simulink model "ARI_24_9_DBtracking"  (Simulink 7.8)
settings: Solver=ode45  SolverMode=SingleTasking  StartTime=0.0  StopTime=20  RelTol=1e-10  AbsTol=1e-10
values from neighbouring files (symbols this model uses):
  h = findobj(gcf,'type','line')    [boldLines.m]    (also in phase.m = min(hmax, 0.9*h*(tau/delta)^pow))
  p = plot(x,y,'b.',0,0,'g*','EraseMode','none','MarkerSize',10);hold on    [PAplot.m]
undefined symbols (not defined in the file or in its folder): A, B, C, D
libraries: simulink x9
settings Model: Creator=Michael Sebek  ModifiedByFormat=Michael Sebek  LastModifiedBy=Michael Sebek  ExtModeTrigMode=oneshot  ExtModeArmWhenConnect=off
settings DataIOCC: LimitDataPoints=off
settings OptimizationCC: BlockReduction=off  BooleanDataType=off  InitFltsAndDblsToZero=on
settings DebuggingCC: SaveWithParameterizedLinksMsg=none  SignalResolutionControl=TryResolveAllWithWarning  SolverPrmCheckMsg=none  MultiTaskDSMMsg=warning  MultiTaskCondExecSysMsg=none  FcnCallInpInsideContextMsg=Use local settings  StrictBusMsg=None
settings HardwareCC: TargetUnknown=on
settings RTWCC: IncludeERTFirstTime=on
settings GRTTargetCC: TargetFcnLib=ansi_tfl_tmw.mat

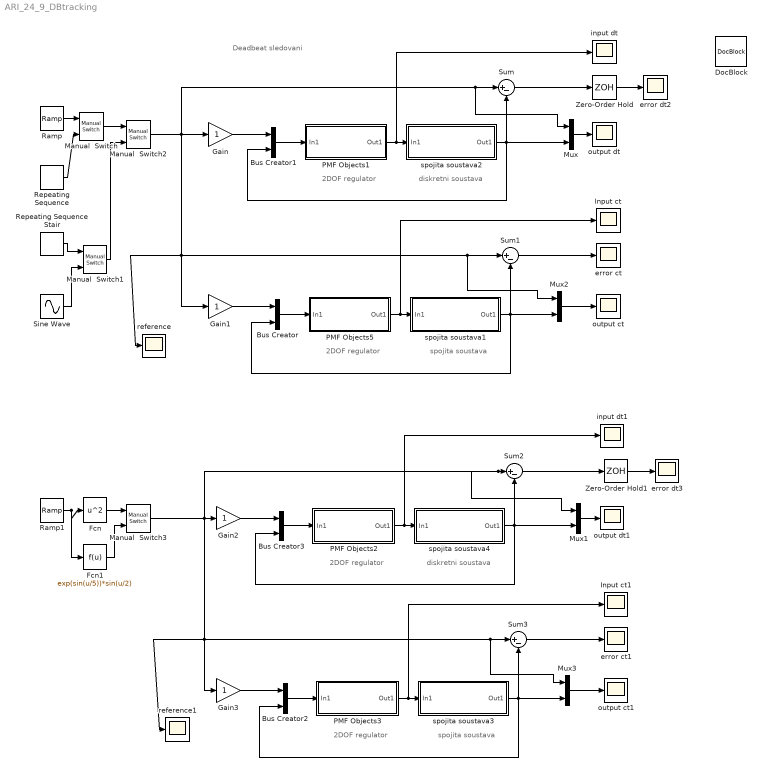
== system ARI_24_9_DBtracking ==
  note: Deadbeat sledovani
  note: spojita soustava
  note: 2DOF regulator
  note: diskretni soustava
  note: 2DOF regulator
  note: spojita soustava
  note: 2DOF regulator
  note: diskretni soustava
  note: 2DOF regulator
  Bus Creator{,1..3} (4 alike) : BusCreator  Inputs=2
  DocBlock : simulink/Model-Wide Utilities/DocBlock  DocumentType=Text
      content=|
      | %%%%%%%%%%%%%%%%%%%%%%%%%%%
      | sledovani rampy
      | %%%%%%%%%%%%%%%%%%%%%%%%%%%
      | h=0.5; m=1;f=(1-zi)^2;
      | a=(1-zi)^2;b=h^2/2*(zi+1)*zi;
      | [p,q]=axbyc(a,b,m);
      | [t,r]=axbyc(f,b,m);
      | p,q,t,r
      |
      | %%%%%%%%%%%%%%%%%%%%%%%%%%%
      | sledovani paraboly
      | %%%%%%%%%%%%%%%%%%%%%%%%%%%
      | h=0.5; m=1;f=(1-zi)^3;
      | a=(1-zi)^2;b=h^2/2*(zi+1)*zi;
      | [p,q]=axbyc(a,b,m);
      | [t,r]=axbyc(f,b,m);
      | p,q,t,r
  Fcn : Fcn  Expr=u^2
  Fcn1 : Fcn  Expr=exp(sin(u/5))*sin(u/2)
  Gain : Gain  SampleTime=h
  Gain1 : Gain
  Gain2 : Gain  SampleTime=h
  Gain3 : Gain
  Input ct : Scope
      settings: TickLabels=on  TimeRange=2  YMin=-2000  YMax=2000  DataFormat=Array
  Input ct1 : Scope
      settings: TickLabels=on  TimeRange=2  YMin=-2000  YMax=2000  SaveName=ScopeData7  DataFormat=Array
  Manual  Switch : simulink/Signal Routing/Manual Switch  sw=1  action=0  varsize=off
  Manual  Switch1 : simulink/Signal Routing/Manual Switch  sw=0  action=0  varsize=off
  Manual  Switch2 : simulink/Signal Routing/Manual Switch  sw=1  action=0  varsize=off
  Manual  Switch3 : simulink/Signal Routing/Manual Switch  sw=1  action=0  varsize=off
  Mux{,1..3} (4 alike) : Mux  Inputs=2
  PMF Objects1 : Subsystem  mask(PMF Block){F=[r -q]/p, InCon=[ ], SampTime=h, fvar=No change}
      mask prompts: F "PMF Object:"; InCon "Initial states:"; SampTime "Sample time (discrete time only):"; fvar "Force variable:"
      mask help:
      | Polynomial matrix fraction description of a linear system.
      |
      | This block represents a linear system defined by the polynomial matrix fraction of its transfer function.
      mask init:
      | Label = 'xxx';
      | [A,B,C,D,Label,var] = polymask2(F, fvar, length(InCon));
      | update;
      mask Help:
      | This block represents a linear system [<I>A,B,C,D</I>] defined by the polynomial matrix fraction (<I>PMF</I>) of its transfer function <I>T</I>.
      | <p>
      | <b>Left Matrix Fraction</b> item of the popup menu <b>Type</b> indicates the transfer function in the form of <I>left PMF</I>:
      | <p>
      | <I>T</I> = inv(<I>Q</I>) <I>P</I>.
      | <p>
      | <b>Right Matrix Fraction</b> item is used if the transfer function is given in the form of <I>right PMF</I>:
      | <p>
      | <I>T</I> = <I>P</I> inv(<I>Q</I>).
      | <p>
      |  The <b>variable</b> determines the type  of the system:
      | <p>
      | - <b>s, p</b> are used for continous time systems (Laplace transform).
      | <p>
      | - <b>z, q</b> are used for discrete time transfer functions in forward-shift operator (Z-transform).
      | <p>
      | - <b>d, z^-1</b> are used for discrete time transfer functions in backward-shift operator.
      | <p>
      | <b> Note:</b> For the variables <I>s,p,z,q</I>, the transfer function is defined as
      | <p>
      | <I>T</I> = <I>C</I> inv(<I>vI-A</I>) <I>B</I> + <I>D</I>,
      | <p>
      | where <I>v</I> is the variable of <I>P,Q</I>.
      | For the variables <I>d, z^-1</I>, the transfer function is defined as
      | <p>
      | <I>T</I> = <I>C v</I> inv(<I>I-Av</I>)  <I>B</I> + <I>D</I>.
      | <p>
      | <b>Note:</b> <b>Initial states</b> concern the observer-form realization of the system as defined by LMF2S and RMF2S functions. Their number must equal the sum of column degrees of the denominator matrix <I>Q</I> in case of right PMF and the sum of row degrees of <I>Q</I> for left PMF description.
      | <p>
      | See also POL, LMF2S, RMF2S.
      mask StyleString: edit,edit,edit,popup(No change|s   (continous time)|p   (continous time)|z      (discrete time)|q      (discrete time)|d      (discrete time)|z^-1 (discrete time))
      mask Display: disp(Label);
  PMF Objects2 : Subsystem  mask(PMF Block){F=[r -q]/p, InCon=[ ], SampTime=h, fvar=No change}
      mask prompts: F "PMF Object:"; InCon "Initial states:"; SampTime "Sample time (discrete time only):"; fvar "Force variable:"
      mask help:
      | Polynomial matrix fraction description of a linear system.
      |
      | This block represents a linear system defined by the polynomial matrix fraction of its transfer function.
      mask init:
      | Label = 'xxx';
      | [A,B,C,D,Label,var] = polymask2(F, fvar, length(InCon));
      | update;
      mask Help:
      | This block represents a linear system [<I>A,B,C,D</I>] defined by the polynomial matrix fraction (<I>PMF</I>) of its transfer function <I>T</I>.
      | <p>
      | <b>Left Matrix Fraction</b> item of the popup menu <b>Type</b> indicates the transfer function in the form of <I>left PMF</I>:
      | <p>
      | <I>T</I> = inv(<I>Q</I>) <I>P</I>.
      | <p>
      | <b>Right Matrix Fraction</b> item is used if the transfer function is given in the form of <I>right PMF</I>:
      | <p>
      | <I>T</I> = <I>P</I> inv(<I>Q</I>).
      | <p>
      |  The <b>variable</b> determines the type  of the system:
      | <p>
      | - <b>s, p</b> are used for continous time systems (Laplace transform).
      | <p>
      | - <b>z, q</b> are used for discrete time transfer functions in forward-shift operator (Z-transform).
      | <p>
      | - <b>d, z^-1</b> are used for discrete time transfer functions in backward-shift operator.
      | <p>
      | <b> Note:</b> For the variables <I>s,p,z,q</I>, the transfer function is defined as
      | <p>
      | <I>T</I> = <I>C</I> inv(<I>vI-A</I>) <I>B</I> + <I>D</I>,
      | <p>
      | where <I>v</I> is the variable of <I>P,Q</I>.
      | For the variables <I>d, z^-1</I>, the transfer function is defined as
      | <p>
      | <I>T</I> = <I>C v</I> inv(<I>I-Av</I>)  <I>B</I> + <I>D</I>.
      | <p>
      | <b>Note:</b> <b>Initial states</b> concern the observer-form realization of the system as defined by LMF2S and RMF2S functions. Their number must equal the sum of column degrees of the denominator matrix <I>Q</I> in case of right PMF and the sum of row degrees of <I>Q</I> for left PMF description.
      | <p>
      | See also POL, LMF2S, RMF2S.
      mask StyleString: edit,edit,edit,popup(No change|s   (continous time)|p   (continous time)|z      (discrete time)|q      (discrete time)|d      (discrete time)|z^-1 (discrete time))
      mask Display: disp(Label);
  PMF Objects3 : Subsystem  mask(PMF Block){F=[r -q]/p, InCon=[ ], SampTime=h, fvar=No change}
      mask prompts: F "PMF Object:"; InCon "Initial states:"; SampTime "Sample time (discrete time only):"; fvar "Force variable:"
      mask help:
      | Polynomial matrix fraction description of a linear system.
      |
      | This block represents a linear system defined by the polynomial matrix fraction of its transfer function.
      mask init:
      | Label = 'xxx';
      | [A,B,C,D,Label,var] = polymask2(F, fvar, length(InCon));
      | update;
      mask Help:
      | This block represents a linear system [<I>A,B,C,D</I>] defined by the polynomial matrix fraction (<I>PMF</I>) of its transfer function <I>T</I>.
      | <p>
      | <b>Left Matrix Fraction</b> item of the popup menu <b>Type</b> indicates the transfer function in the form of <I>left PMF</I>:
      | <p>
      | <I>T</I> = inv(<I>Q</I>) <I>P</I>.
      | <p>
      | <b>Right Matrix Fraction</b> item is used if the transfer function is given in the form of <I>right PMF</I>:
      | <p>
      | <I>T</I> = <I>P</I> inv(<I>Q</I>).
      | <p>
      |  The <b>variable</b> determines the type  of the system:
      | <p>
      | - <b>s, p</b> are used for continous time systems (Laplace transform).
      | <p>
      | - <b>z, q</b> are used for discrete time transfer functions in forward-shift operator (Z-transform).
      | <p>
      | - <b>d, z^-1</b> are used for discrete time transfer functions in backward-shift operator.
      | <p>
      | <b> Note:</b> For the variables <I>s,p,z,q</I>, the transfer function is defined as
      | <p>
      | <I>T</I> = <I>C</I> inv(<I>vI-A</I>) <I>B</I> + <I>D</I>,
      | <p>
      | where <I>v</I> is the variable of <I>P,Q</I>.
      | For the variables <I>d, z^-1</I>, the transfer function is defined as
      | <p>
      | <I>T</I> = <I>C v</I> inv(<I>I-Av</I>)  <I>B</I> + <I>D</I>.
      | <p>
      | <b>Note:</b> <b>Initial states</b> concern the observer-form realization of the system as defined by LMF2S and RMF2S functions. Their number must equal the sum of column degrees of the denominator matrix <I>Q</I> in case of right PMF and the sum of row degrees of <I>Q</I> for left PMF description.
      | <p>
      | See also POL, LMF2S, RMF2S.
      mask StyleString: edit,edit,edit,popup(No change|s   (continous time)|p   (continous time)|z      (discrete time)|q      (discrete time)|d      (discrete time)|z^-1 (discrete time))
      mask Display: disp(Label);
  PMF Objects5 : Subsystem  mask(PMF Block){F=[r -q]/p, InCon=[ ], SampTime=h, fvar=No change}
      mask prompts: F "PMF Object:"; InCon "Initial states:"; SampTime "Sample time (discrete time only):"; fvar "Force variable:"
      mask help:
      | Polynomial matrix fraction description of a linear system.
      |
      | This block represents a linear system defined by the polynomial matrix fraction of its transfer function.
      mask init:
      | Label = 'xxx';
      | [A,B,C,D,Label,var] = polymask2(F, fvar, length(InCon));
      | update;
      mask Help:
      | This block represents a linear system [<I>A,B,C,D</I>] defined by the polynomial matrix fraction (<I>PMF</I>) of its transfer function <I>T</I>.
      | <p>
      | <b>Left Matrix Fraction</b> item of the popup menu <b>Type</b> indicates the transfer function in the form of <I>left PMF</I>:
      | <p>
      | <I>T</I> = inv(<I>Q</I>) <I>P</I>.
      | <p>
      | <b>Right Matrix Fraction</b> item is used if the transfer function is given in the form of <I>right PMF</I>:
      | <p>
      | <I>T</I> = <I>P</I> inv(<I>Q</I>).
      | <p>
      |  The <b>variable</b> determines the type  of the system:
      | <p>
      | - <b>s, p</b> are used for continous time systems (Laplace transform).
      | <p>
      | - <b>z, q</b> are used for discrete time transfer functions in forward-shift operator (Z-transform).
      | <p>
      | - <b>d, z^-1</b> are used for discrete time transfer functions in backward-shift operator.
      | <p>
      | <b> Note:</b> For the variables <I>s,p,z,q</I>, the transfer function is defined as
      | <p>
      | <I>T</I> = <I>C</I> inv(<I>vI-A</I>) <I>B</I> + <I>D</I>,
      | <p>
      | where <I>v</I> is the variable of <I>P,Q</I>.
      | For the variables <I>d, z^-1</I>, the transfer function is defined as
      | <p>
      | <I>T</I> = <I>C v</I> inv(<I>I-Av</I>)  <I>B</I> + <I>D</I>.
      | <p>
      | <b>Note:</b> <b>Initial states</b> concern the observer-form realization of the system as defined by LMF2S and RMF2S functions. Their number must equal the sum of column degrees of the denominator matrix <I>Q</I> in case of right PMF and the sum of row degrees of <I>Q</I> for left PMF description.
      | <p>
      | See also POL, LMF2S, RMF2S.
      mask StyleString: edit,edit,edit,popup(No change|s   (continous time)|p   (continous time)|z      (discrete time)|q      (discrete time)|d      (discrete time)|z^-1 (discrete time))
      mask Display: disp(Label);
  Ramp : simulink/Sources/Ramp  slope=1  start=0  X0=0
  Ramp1 : simulink/Sources/Ramp  slope=1  start=0  X0=0
  Repeating Sequence : simulink/Sources/Repeating Sequence  rep_seq_t=[0 8]  rep_seq_y=[0 5]
  Repeating Sequence Stair : simulink/Sources/Repeating Sequence Stair  OutValues="[3 1  4 2   1].'"  tsamp=10  OutMin=[]  OutMax=[]  OutDataTypeStr=float('double')  OutputDataTypeScalingMode=Specify via dialog  OutDataType=float('double')  ConRadixGroup=Best Precision: Vector-wise  OutScaling=2^-12
  Sine Wave : Sin  Frequency=.5  SampleTime=0
  Sum{,1..3} (4 alike) : Sum  Inputs=|+-
  Zero-Order Hold : ZeroOrderHold  SampleTime=h
  Zero-Order Hold1 : ZeroOrderHold  SampleTime=h
  error ct : Scope
      settings: TickLabels=on  TimeRange=2  YMin=-2000  YMax=2000  SaveName=ScopeData5  DataFormat=Array
  error ct1 : Scope
      settings: TickLabels=on  TimeRange=2  YMin=-2000  YMax=2000  SaveName=ScopeData8  DataFormat=Array
  error dt2 : Scope
      settings: TickLabels=on  TimeRange=2  YMin=-2000  YMax=2000  SaveName=ScopeData14  DataFormat=Array
  error dt3 : Scope
      settings: TickLabels=on  TimeRange=2  YMin=-2000  YMax=2000  SaveName=ScopeData15  DataFormat=Array
  input dt : Scope
      settings: TickLabels=on  TimeRange=2  YMin=-2000  YMax=2000  DataFormat=Array
  input dt1 : Scope
      settings: TickLabels=on  TimeRange=2  YMin=-2000  YMax=2000  SaveName=ScopeData10  DataFormat=Array
  output ct : Scope
      settings: TickLabels=on  TimeRange=2  YMin=-1  YMax=3  SaveName=ScopeData2  DataFormat=Array
  output ct1 : Scope
      settings: TickLabels=on  TimeRange=2  YMin=-1  YMax=3  SaveName=ScopeData11  DataFormat=Array
  output dt : Scope
      settings: TickLabels=on  TimeRange=2  YMin=-1  YMax=3  SaveName=ScopeData3  DataFormat=Array
  output dt1 : Scope
      settings: TickLabels=on  TimeRange=2  YMin=-1  YMax=3  SaveName=ScopeData12  DataFormat=Array
  reference : Scope
      settings: TickLabels=on  TimeRange=2  YMin=-2000  YMax=2000  SaveName=ScopeData6  DataFormat=Array
  reference1 : Scope
      settings: TickLabels=on  TimeRange=2  YMin=-2000  YMax=2000  SaveName=ScopeData13  DataFormat=Array
  spojita soustava1 : Subsystem  mask(PMF Block){F=1/s^2, InCon=[ ], SampTime=h, fvar=No change}
      mask prompts: F "PMF Object:"; InCon "Initial states:"; SampTime "Sample time (discrete time only):"; fvar "Force variable:"
      mask help:
      | Polynomial matrix fraction description of a linear system.
      |
      | This block represents a linear system defined by the polynomial matrix fraction of its transfer function.
      mask init:
      | Label = 'xxx';
      | [A,B,C,D,Label,var] = polymask2(F, fvar, length(InCon));
      | update;
      mask Help:
      | This block represents a linear system [<I>A,B,C,D</I>] defined by the polynomial matrix fraction (<I>PMF</I>) of its transfer function <I>T</I>.
      | <p>
      | <b>Left Matrix Fraction</b> item of the popup menu <b>Type</b> indicates the transfer function in the form of <I>left PMF</I>:
      | <p>
      | <I>T</I> = inv(<I>Q</I>) <I>P</I>.
      | <p>
      | <b>Right Matrix Fraction</b> item is used if the transfer function is given in the form of <I>right PMF</I>:
      | <p>
      | <I>T</I> = <I>P</I> inv(<I>Q</I>).
      | <p>
      |  The <b>variable</b> determines the type  of the system:
      | <p>
      | - <b>s, p</b> are used for continous time systems (Laplace transform).
      | <p>
      | - <b>z, q</b> are used for discrete time transfer functions in forward-shift operator (Z-transform).
      | <p>
      | - <b>d, z^-1</b> are used for discrete time transfer functions in backward-shift operator.
      | <p>
      | <b> Note:</b> For the variables <I>s,p,z,q</I>, the transfer function is defined as
      | <p>
      | <I>T</I> = <I>C</I> inv(<I>vI-A</I>) <I>B</I> + <I>D</I>,
      | <p>
      | where <I>v</I> is the variable of <I>P,Q</I>.
      | For the variables <I>d, z^-1</I>, the transfer function is defined as
      | <p>
      | <I>T</I> = <I>C v</I> inv(<I>I-Av</I>)  <I>B</I> + <I>D</I>.
      | <p>
      | <b>Note:</b> <b>Initial states</b> concern the observer-form realization of the system as defined by LMF2S and RMF2S functions. Their number must equal the sum of column degrees of the denominator matrix <I>Q</I> in case of right PMF and the sum of row degrees of <I>Q</I> for left PMF description.
      | <p>
      | See also POL, LMF2S, RMF2S.
      mask StyleString: edit,edit,edit,popup(No change|s   (continous time)|p   (continous time)|z      (discrete time)|q      (discrete time)|d      (discrete time)|z^-1 (discrete time))
      mask Display: disp(Label);
  spojita soustava2 : Subsystem  mask(PMF Block){F=b/a, InCon=[ ], SampTime=h, fvar=No change}
      mask prompts: F "PMF Object:"; InCon "Initial states:"; SampTime "Sample time (discrete time only):"; fvar "Force variable:"
      mask help:
      | Polynomial matrix fraction description of a linear system.
      |
      | This block represents a linear system defined by the polynomial matrix fraction of its transfer function.
      mask init:
      | Label = 'xxx';
      | [A,B,C,D,Label,var] = polymask2(F, fvar, length(InCon));
      | update;
      mask Help:
      | This block represents a linear system [<I>A,B,C,D</I>] defined by the polynomial matrix fraction (<I>PMF</I>) of its transfer function <I>T</I>.
      | <p>
      | <b>Left Matrix Fraction</b> item of the popup menu <b>Type</b> indicates the transfer function in the form of <I>left PMF</I>:
      | <p>
      | <I>T</I> = inv(<I>Q</I>) <I>P</I>.
      | <p>
      | <b>Right Matrix Fraction</b> item is used if the transfer function is given in the form of <I>right PMF</I>:
      | <p>
      | <I>T</I> = <I>P</I> inv(<I>Q</I>).
      | <p>
      |  The <b>variable</b> determines the type  of the system:
      | <p>
      | - <b>s, p</b> are used for continous time systems (Laplace transform).
      | <p>
      | - <b>z, q</b> are used for discrete time transfer functions in forward-shift operator (Z-transform).
      | <p>
      | - <b>d, z^-1</b> are used for discrete time transfer functions in backward-shift operator.
      | <p>
      | <b> Note:</b> For the variables <I>s,p,z,q</I>, the transfer function is defined as
      | <p>
      | <I>T</I> = <I>C</I> inv(<I>vI-A</I>) <I>B</I> + <I>D</I>,
      | <p>
      | where <I>v</I> is the variable of <I>P,Q</I>.
      | For the variables <I>d, z^-1</I>, the transfer function is defined as
      | <p>
      | <I>T</I> = <I>C v</I> inv(<I>I-Av</I>)  <I>B</I> + <I>D</I>.
      | <p>
      | <b>Note:</b> <b>Initial states</b> concern the observer-form realization of the system as defined by LMF2S and RMF2S functions. Their number must equal the sum of column degrees of the denominator matrix <I>Q</I> in case of right PMF and the sum of row degrees of <I>Q</I> for left PMF description.
      | <p>
      | See also POL, LMF2S, RMF2S.
      mask StyleString: edit,edit,edit,popup(No change|s   (continous time)|p   (continous time)|z      (discrete time)|q      (discrete time)|d      (discrete time)|z^-1 (discrete time))
      mask Display: disp(Label);
  spojita soustava3 : Subsystem  mask(PMF Block){F=1/s^2, InCon=[ ], SampTime=h, fvar=No change}
      mask prompts: F "PMF Object:"; InCon "Initial states:"; SampTime "Sample time (discrete time only):"; fvar "Force variable:"
      mask help:
      | Polynomial matrix fraction description of a linear system.
      |
      | This block represents a linear system defined by the polynomial matrix fraction of its transfer function.
      mask init:
      | Label = 'xxx';
      | [A,B,C,D,Label,var] = polymask2(F, fvar, length(InCon));
      | update;
      mask Help:
      | This block represents a linear system [<I>A,B,C,D</I>] defined by the polynomial matrix fraction (<I>PMF</I>) of its transfer function <I>T</I>.
      | <p>
      | <b>Left Matrix Fraction</b> item of the popup menu <b>Type</b> indicates the transfer function in the form of <I>left PMF</I>:
      | <p>
      | <I>T</I> = inv(<I>Q</I>) <I>P</I>.
      | <p>
      | <b>Right Matrix Fraction</b> item is used if the transfer function is given in the form of <I>right PMF</I>:
      | <p>
      | <I>T</I> = <I>P</I> inv(<I>Q</I>).
      | <p>
      |  The <b>variable</b> determines the type  of the system:
      | <p>
      | - <b>s, p</b> are used for continous time systems (Laplace transform).
      | <p>
      | - <b>z, q</b> are used for discrete time transfer functions in forward-shift operator (Z-transform).
      | <p>
      | - <b>d, z^-1</b> are used for discrete time transfer functions in backward-shift operator.
      | <p>
      | <b> Note:</b> For the variables <I>s,p,z,q</I>, the transfer function is defined as
      | <p>
      | <I>T</I> = <I>C</I> inv(<I>vI-A</I>) <I>B</I> + <I>D</I>,
      | <p>
      | where <I>v</I> is the variable of <I>P,Q</I>.
      | For the variables <I>d, z^-1</I>, the transfer function is defined as
      | <p>
      | <I>T</I> = <I>C v</I> inv(<I>I-Av</I>)  <I>B</I> + <I>D</I>.
      | <p>
      | <b>Note:</b> <b>Initial states</b> concern the observer-form realization of the system as defined by LMF2S and RMF2S functions. Their number must equal the sum of column degrees of the denominator matrix <I>Q</I> in case of right PMF and the sum of row degrees of <I>Q</I> for left PMF description.
      | <p>
      | See also POL, LMF2S, RMF2S.
      mask StyleString: edit,edit,edit,popup(No change|s   (continous time)|p   (continous time)|z      (discrete time)|q      (discrete time)|d      (discrete time)|z^-1 (discrete time))
      mask Display: disp(Label);
  spojita soustava4 : Subsystem  mask(PMF Block){F=b/a, InCon=[ ], SampTime=h, fvar=No change}
      mask prompts: F "PMF Object:"; InCon "Initial states:"; SampTime "Sample time (discrete time only):"; fvar "Force variable:"
      mask help:
      | Polynomial matrix fraction description of a linear system.
      |
      | This block represents a linear system defined by the polynomial matrix fraction of its transfer function.
      mask init:
      | Label = 'xxx';
      | [A,B,C,D,Label,var] = polymask2(F, fvar, length(InCon));
      | update;
      mask Help:
      | This block represents a linear system [<I>A,B,C,D</I>] defined by the polynomial matrix fraction (<I>PMF</I>) of its transfer function <I>T</I>.
      | <p>
      | <b>Left Matrix Fraction</b> item of the popup menu <b>Type</b> indicates the transfer function in the form of <I>left PMF</I>:
      | <p>
      | <I>T</I> = inv(<I>Q</I>) <I>P</I>.
      | <p>
      | <b>Right Matrix Fraction</b> item is used if the transfer function is given in the form of <I>right PMF</I>:
      | <p>
      | <I>T</I> = <I>P</I> inv(<I>Q</I>).
      | <p>
      |  The <b>variable</b> determines the type  of the system:
      | <p>
      | - <b>s, p</b> are used for continous time systems (Laplace transform).
      | <p>
      | - <b>z, q</b> are used for discrete time transfer functions in forward-shift operator (Z-transform).
      | <p>
      | - <b>d, z^-1</b> are used for discrete time transfer functions in backward-shift operator.
      | <p>
      | <b> Note:</b> For the variables <I>s,p,z,q</I>, the transfer function is defined as
      | <p>
      | <I>T</I> = <I>C</I> inv(<I>vI-A</I>) <I>B</I> + <I>D</I>,
      | <p>
      | where <I>v</I> is the variable of <I>P,Q</I>.
      | For the variables <I>d, z^-1</I>, the transfer function is defined as
      | <p>
      | <I>T</I> = <I>C v</I> inv(<I>I-Av</I>)  <I>B</I> + <I>D</I>.
      | <p>
      | <b>Note:</b> <b>Initial states</b> concern the observer-form realization of the system as defined by LMF2S and RMF2S functions. Their number must equal the sum of column degrees of the denominator matrix <I>Q</I> in case of right PMF and the sum of row degrees of <I>Q</I> for left PMF description.
      | <p>
      | See also POL, LMF2S, RMF2S.
      mask StyleString: edit,edit,edit,popup(No change|s   (continous time)|p   (continous time)|z      (discrete time)|q      (discrete time)|d      (discrete time)|z^-1 (discrete time))
      mask Display: disp(Label);
  wires:
  spojita soustava1/1(Out1) -> Bus Creator/2, Sum1/2, Mux2/2
  Mux2/1 -> output ct/1
  Gain1/1 -> Bus Creator/1
  Bus Creator/1 -> PMF Objects5/1(In1)
  PMF Objects5/1(Out1) -> spojita soustava1/1(In1), Input ct/1
  spojita soustava2/1(Out1) -> Sum/2, Mux/2, Bus Creator1/2
  Gain/1 -> Bus Creator1/1
  Bus Creator1/1 -> PMF Objects1/1(In1)
  PMF Objects1/1(Out1) -> input dt/1, spojita soustava2/1(In1)
  Sum/1 -> Zero-Order Hold/1
  Ramp/1 -> Manual  Switch/1
  Repeating Sequence/1 -> Manual  Switch/2
  Mux/1 -> output dt/1
  Sum1/1 -> error ct/1
  Manual  Switch/1 -> Manual  Switch2/1
  Manual  Switch2/1 -> Gain/1, Gain1/1, Sum1/1, Mux2/1, reference/1, Sum/1, Mux/1
  Manual  Switch1/1 -> Manual  Switch2/2
  Repeating Sequence Stair/1 -> Manual  Switch1/1
  Sine Wave/1 -> Manual  Switch1/2
  spojita soustava3/1(Out1) -> Bus Creator2/2, Sum3/2, Mux3/2
  Mux3/1 -> output ct1/1
  Gain3/1 -> Bus Creator2/1
  Bus Creator2/1 -> PMF Objects3/1(In1)
  PMF Objects3/1(Out1) -> spojita soustava3/1(In1), Input ct1/1
  spojita soustava4/1(Out1) -> Bus Creator3/2, Sum2/2, Mux1/2
  Gain2/1 -> Bus Creator3/1
  Bus Creator3/1 -> PMF Objects2/1(In1)
  PMF Objects2/1(Out1) -> input dt1/1, spojita soustava4/1(In1)
  Sum2/1 -> Zero-Order Hold1/1
  Fcn/1 -> Manual  Switch3/1
  Fcn1/1 -> Manual  Switch3/2
  Mux1/1 -> output dt1/1
  Sum3/1 -> error ct1/1
  Manual  Switch3/1 -> Gain2/1, Gain3/1, Sum3/1, Mux3/1, reference1/1, Sum2/1, Mux1/1
  Ramp1/1 -> Fcn1/1, Fcn/1
  Zero-Order Hold/1 -> error dt2/1
  Zero-Order Hold1/1 -> error dt3/1

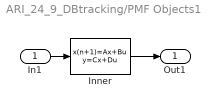
== system ARI_24_9_DBtracking/PMF Objects1 ==
  In1 : Inport
  Inner : DiscreteStateSpace  A=A  B=B  C=C  D=D  X0=InCon  SampleTime=SampTime
  Out1 : Outport
  wires:
  In1/1 -> Inner/1
  Inner/1 -> Out1/1

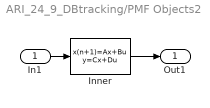
== system ARI_24_9_DBtracking/PMF Objects2 ==
  In1 : Inport
  Inner : DiscreteStateSpace  A=A  B=B  C=C  D=D  X0=InCon  SampleTime=SampTime
  Out1 : Outport
  wires:
  In1/1 -> Inner/1
  Inner/1 -> Out1/1

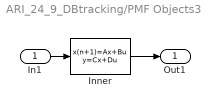
== system ARI_24_9_DBtracking/PMF Objects3 ==
  In1 : Inport
  Inner : DiscreteStateSpace  A=A  B=B  C=C  D=D  X0=InCon  SampleTime=SampTime
  Out1 : Outport
  wires:
  Inner/1 -> Out1/1
  In1/1 -> Inner/1

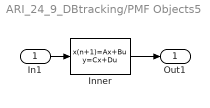
== system ARI_24_9_DBtracking/PMF Objects5 ==
  In1 : Inport
  Inner : DiscreteStateSpace  A=A  B=B  C=C  D=D  X0=InCon  SampleTime=SampTime
  Out1 : Outport
  wires:
  Inner/1 -> Out1/1
  In1/1 -> Inner/1

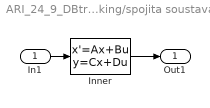
== system ARI_24_9_DBtracking/spojita soustava1 ==
  In1 : Inport
  Inner : StateSpace  A=A  B=B  C=C  D=D  X0=InCon
  Out1 : Outport
  wires:
  In1/1 -> Inner/1
  Inner/1 -> Out1/1

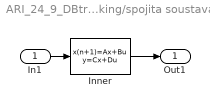
== system ARI_24_9_DBtracking/spojita soustava2 ==
  In1 : Inport
  Inner : DiscreteStateSpace  A=A  B=B  C=C  D=D  X0=InCon  SampleTime=SampTime
  Out1 : Outport
  wires:
  Inner/1 -> Out1/1
  In1/1 -> Inner/1

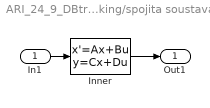
== system ARI_24_9_DBtracking/spojita soustava3 ==
  In1 : Inport
  Inner : StateSpace  A=A  B=B  C=C  D=D  X0=InCon
  Out1 : Outport
  wires:
  In1/1 -> Inner/1
  Inner/1 -> Out1/1

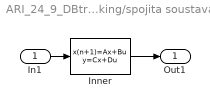
== system ARI_24_9_DBtracking/spojita soustava4 ==
  In1 : Inport
  Inner : DiscreteStateSpace  A=A  B=B  C=C  D=D  X0=InCon  SampleTime=SampTime
  Out1 : Outport
  wires:
  Inner/1 -> Out1/1
  In1/1 -> Inner/1
